simulink model "motor"  (R2013b)
settings: Solver=FixedStepDiscrete  SolverMode=SingleTasking  StartTime=0.0  StopTime=inf  RelTol=1e-3
libraries: embdlinuxlib x6
settings Model: SimulationMode=external  ExtModeTrigDuration=100  Creator=Lester  LastModifiedBy=Lester
settings OptimizationCC: OptimizeModelRefInitCode=on  LifeSpan=1
settings DebuggingCC: SolverPrmCheckMsg=none
settings HardwareCC: ProdLargestAtomicInteger=Long  ProdLargestAtomicFloat=Double  ProdEndianess=LittleEndian  ProdHWDeviceType=ARM Compatible->ARM Cortex
settings RTWCC: SystemTargetFile=realtime.tlc  GenerateMakefile=off  TemplateMakefile=realtime.tmf  Description=Run on Target Hardware  RTWVerbose=off  ProcessScript=realtime_make_rtw_hook
settings STFCustomTargetCC: TargetLibSuffix=.a  GenerateSampleERTMain=on  ERTCustomFileBanners=on  SupportNonInlinedSFcns=off  SupportVariableSizeSignals=on  MATLABClassNameForMDSCustomization=Simulink.SoftwareTarget.ERTCustomization  GRTInterface=off  SystemTargetFile=realtime.tlc
settings ERTTargetCC: CodeReplacementLibrary=ANSI_C  GenerateSampleERTMain=on  ParMdlRefBuildCompliant=off  CompOptLevelCompliant=off  ConcurrentExecutionCompliant=off  CombineOutputUpdateFcns=off  ERTFirstTimeCompliant=off  SupportContinuousTime=on  SupportVariableSizeSignals=on  ModelStepFunctionPrototypeControlCompliant=off  CPPClassGenCompliant=off  ExtModeMexArgs='169.254.0.2' 0 17725  InlinedParameterPlacement=NonHierarchical  ERTSrcFileBannerTemplate=realtime_code_template.cgt  ERTHdrFileBannerTemplate=realtime_code_template.cgt  ERTDataSrcFileTemplate=realtime_code_template.cgt  ERTDataHdrFileTemplate=realtime_code_template.cgt  ERTCustomFileTemplate=realtime_file_process.tlc
settings ConfigurationSet: Description=SimMechanics 2G

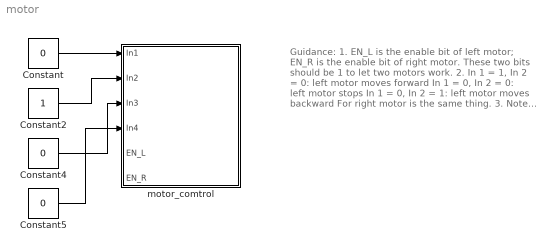
== system motor ==
  note: Guidance:
      | 1. EN_L is the enable bit of left motor;
      | EN_R is the enable bit of right motor. These
      | two bits should be 1 to let two motors work.
      | 2. In 1 = 1, In 2 = 0: left motor moves forward
      |     In 1 = 0, In 2 = 0: left motor stops
      |     In 1 = 0, In 2 = 1: left motor moves backward
      |     For right motor is the same thing.
      | 3. Note that all the inputs type should be boolean.
  Constant : Constant  Value=0  OutDataTypeStr=boolean
  Constant2 : Constant  OutDataTypeStr=boolean
  Constant4 : Constant  Value=0  OutDataTypeStr=boolean
  Constant5 : Constant  Value=0  OutDataTypeStr=boolean
  motor_comtrol : Subsystem
  wires:
  Constant/1 -> motor_comtrol/1(In1)
  Constant2/1 -> motor_comtrol/2(In2)
  Constant4/1 -> motor_comtrol/3(In3)
  Constant5/1 -> motor_comtrol/4(In4)

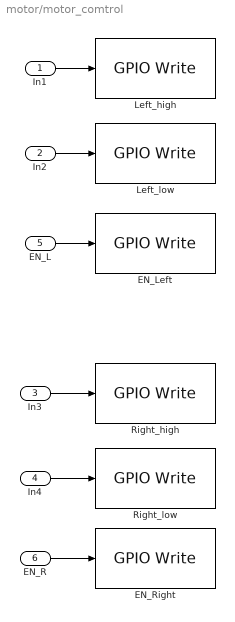
== system motor/motor_comtrol ==
  In1 : Inport
  In2 : Inport  Port=2
  In3 : Inport  Port=3
  In4 : Inport  Port=4
  EN_L : Inport  Port=5
  EN_R : Inport  Port=6
  EN_Left : embdlinuxlib/GPIO Write  board=Model B Rev2  gpio=27  direction=Output  blockPlatform=Raspberry Pi
  EN_Right : embdlinuxlib/GPIO Write  board=Model B Rev2  gpio=22  direction=Output  blockPlatform=Raspberry Pi
  Left_high : embdlinuxlib/GPIO Write  board=Model B Rev2  gpio=4  direction=Output  blockPlatform=Raspberry Pi
  Left_low : embdlinuxlib/GPIO Write  board=Model B Rev2  gpio=17  direction=Output  blockPlatform=Raspberry Pi
  Right_high : embdlinuxlib/GPIO Write  board=Model B Rev2  gpio=23  direction=Output  blockPlatform=Raspberry Pi
  Right_low : embdlinuxlib/GPIO Write  board=Model B Rev2  gpio=24  direction=Output  blockPlatform=Raspberry Pi
  wires:
  In1/1 -> Left_high/1
  In3/1 -> Right_high/1
  In2/1 -> Left_low/1
  In4/1 -> Right_low/1
  EN_L/1 -> EN_Left/1
  EN_R/1 -> EN_Right/1
